simulink model "SIM_BB"  (R2021a)
settings: Solver=VariableStepAuto  StartTime=0.0  StopTime=10  RelTol=1e-3
settings Model: Creator=USER  LastModifiedBy=USER

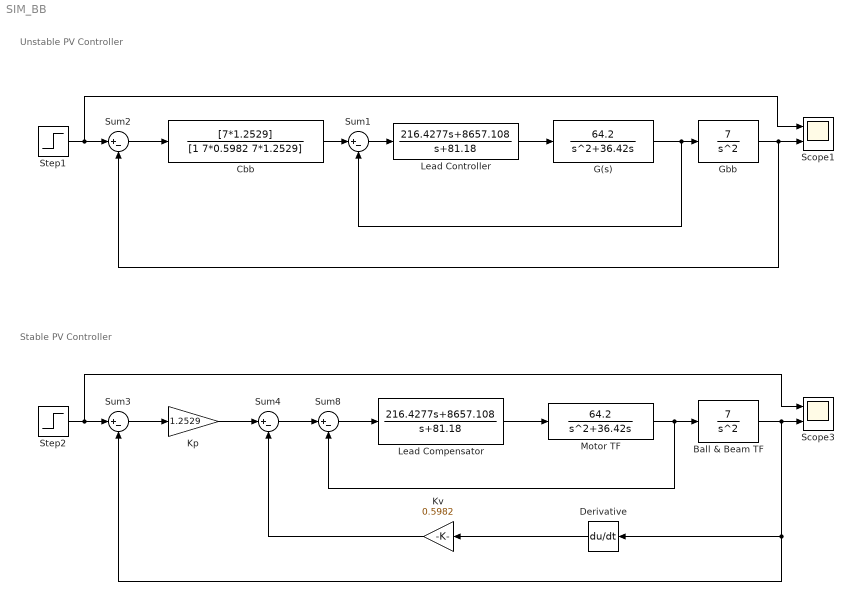
== system SIM_BB ==
  note: Unstable PV Controller
  note: Stable PV Controller
  Ball & Beam TF : TransferFcn  Numerator=[7]  Denominator=[1 0 0]
  Cbb : TransferFcn  Numerator=[7*1.2529]  Denominator=[1 7*0.5982 7*1.2529]
  Derivative : Derivative  CoefficientInTFapproximation=0
  G(s) : TransferFcn  Numerator=[0 64.2]  Denominator=[1 36.42 0]
  Gbb : TransferFcn  Numerator=[7]  Denominator=[1 0 0]
  Kp : Gain  Gain=1.2529
  Kv : Gain  Gain=0.5982
  Lead Compensator : TransferFcn  Numerator=[216.4277 8657.108]  Denominator=[1 81.18]
  Lead Controller : TransferFcn  Numerator=[216.4277 8657.108]  Denominator=[1 81.18]
  Motor TF : TransferFcn  Numerator=[64.2]  Denominator=[1 36.42 0]
  Scope1 : Scope  NumInputPorts=2
  Scope3 : Scope  NumInputPorts=2
  Step1 : Step  Time=0  SampleTime=0
  Step2 : Step  Time=0  SampleTime=0
  Sum{1..4,8} (5 alike) : Sum  Inputs=|+-
  wires:
  Sum1/1 -> Lead Controller/1
  Step1/1 -> Sum2/1, Scope1/1
  Lead Controller/1 -> G(s)/1
  Cbb/1 -> Sum1/1
  Sum2/1 -> Cbb/1
  G(s)/1 -> Sum1/2, Gbb/1
  Gbb/1 -> Sum2/2, Scope1/2
  Motor TF/1 -> Sum8/2, Ball & Beam TF/1
  Lead Compensator/1 -> Motor TF/1
  Sum8/1 -> Lead Compensator/1
  Sum4/1 -> Sum8/1
  Kp/1 -> Sum4/1
  Sum3/1 -> Kp/1
  Step2/1 -> Scope3/1, Sum3/1
  Derivative/1 -> Kv/1
  Kv/1 -> Sum4/2
  Ball & Beam TF/1 -> Scope3/2, Sum3/2, Derivative/1
